simulink model "fuzzyPID0106"  (R2020a)
settings: Solver=VariableStepAuto  StartTime=0.0  StopTime=13  FixedStep=0.01  RelTol=1e-3
libraries: fuzblock x1
settings Model: Creator=chenj  LastModifiedBy=chenj

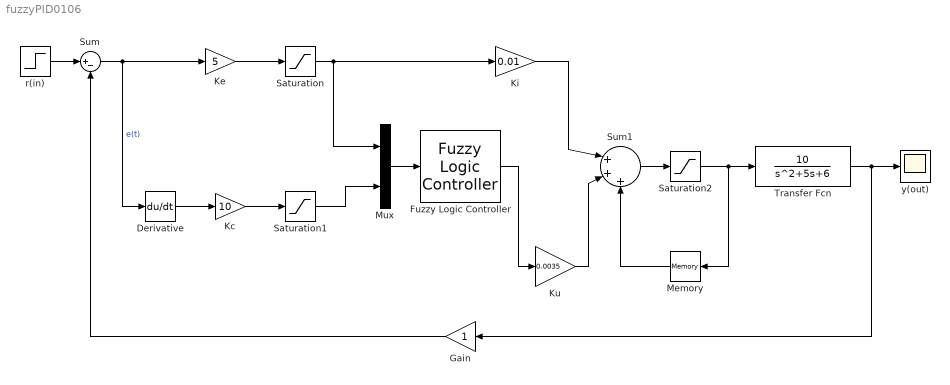
== system fuzzyPID0106 ==
  Derivative : Derivative
  Fuzzy Logic Controller : fuzblock/Fuzzy Logic  Controller  FIS='tipper.fis'  OutputSampleNumber=101  DataType=double  FuzzifiedInputs=off  RuleFiringStrengths=off  RuleOutputs=off  AggregatedOutputs=off  SimulateUsing=Interpreted execution  OutOfRangeInputValueMessage=warning  NoRuleFiredMessage=warning  EmptyOutputFuzzySetMessage=warning
  Gain : Gain
  Kc : Gain  Gain=10
  Ke : Gain  Gain=5
  Ki : Gain  Gain=0.01
  Ku : Gain  Gain=0.0035
  Memory : Memory
  Mux : Mux  Inputs=2
  Saturation : Saturate  UpperLimit=6  LowerLimit=-6
  Saturation1 : Saturate  UpperLimit=6  LowerLimit=-6
  Saturation2 : Saturate  UpperLimit=1  LowerLimit=0
  Sum : Sum  Inputs=|+-
  Sum1 : Sum  Inputs=|+++
  Transfer Fcn : TransferFcn  Numerator=[10]  Denominator=[1 5 6]
  r(in) : Step  After=0.8  SampleTime=0
  y(out) : Scope
  wires:
  Mux/1 -> Fuzzy Logic Controller/1
  r(in)/1 -> Sum/1
  Memory/1 -> Sum1/3
  Saturation2/1 -> Transfer Fcn/1, Memory/1
  Transfer Fcn/1 -> Gain/1, y(out)/1
  Sum1/1 -> Saturation2/1
  Ku/1 -> Sum1/2
  Fuzzy Logic Controller/1 -> Ku/1
  Ki/1 -> Sum1/1
  Saturation/1 -> Ki/1, Mux/1
  Saturation1/1 -> Mux/2
  Kc/1 -> Saturation1/1
  Derivative/1 -> Kc/1
  Ke/1 -> Saturation/1
  Sum/1 -> Derivative/1, Ke/1  "e(t)"
  Gain/1 -> Sum/2
